simulink model "ReferenceTrajectory"  (R2021a)
settings: Solver=VariableStepAuto  StartTime=0.0  StopTime=10.0  RelTol=1e-3
libraries: simulink x1
settings Model: Creator=Davide  LastModifiedBy=Davide

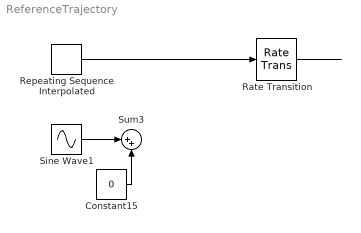
== system ReferenceTrajectory ==
  Constant15 : Constant  Value=0
  Rate Transition : RateTransition  Deterministic=off
  Repeating Sequence Interpolated : simulink/Sources/Repeating Sequence Interpolated  OutValues=[0 800 1000 1000 500 0 0 -500 -500 0].'  TimeValues=[0 0.3 0.5 1 1.2 1.4 1.7 2 2.2 2.5].'  LookUpMeth=Interpolation-Use End Values  tsamp=0.0001  OutMin=[]  OutMax=[]  OutDataTypeStr=double  OutputDataTypeScalingMode=double  OutDataType=fixdt(0,8)  OutScaling=2^-10
  Sine Wave1 : Sin  Amplitude=500  Frequency=15  SampleTime=0.0001
  Sum3 : Sum  Inputs=|++
  wires:
  Sine Wave1/1 -> Sum3/1
  Constant15/1 -> Sum3/2
  Repeating Sequence Interpolated/1 -> Rate Transition/1
  Rate Transition/1 -> ?
